simulink model "dual_arm_1"  (R2021b)
settings: Solver=FixedStepAuto  StartTime=0.0  StopTime=10  FixedStep=0.01  RelTol=1e-3
values from neighbouring files (symbols this model uses):
  a0 = 0.99    [load_main.m]
  b1 = base1.q    [load_main.m]
  b2 = base2.q    [load_main.m]
  berta = 0.98    [load_main.m]
  csi = 0.4    [load_main.m]
  dyr_in = [0 0 0 0 0 0]'    [load_main.m]
  F_int_max = [5;5]    [load_main.m]
  F_max = [1;1]    [load_main.m]
  franka_dh_matrix = [FEp_DH_theta;FEp_DH_d; FEp_DH_a;FEp_DH_alpha]    [load_main.m]
  inc = 1000    [load_main.m]
  mass = 1    [load_main.m]    (also in mod_k.m)
  q_in_1 = [0.4670   -0.1818    0.1521   -2.2022   -2.1767    2.4575    2.3293]    [load_main.m]
  q_in_2 = [-0.4654   -0.1791   -0.1528   -2.1994    2.1769    2.4577   -2.3291]    [load_main.m]
  Ts = 0.01    [load_main.m]
  yr_in = vec6(log(DQ(e_in)))    [load_main.m]
undefined symbols (not defined in the file or in its folder): k_default
settings Model: Creator=rachele  LastModifiedBy=geriatronics
settings SolverCC: AlgebraicLoopSolver=TrustRegion
settings DebuggingCC: SFMachineParentedDataDiag=warning

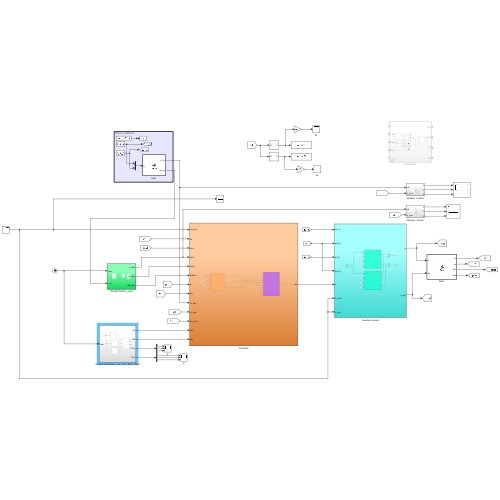
[thumbnail: Simulink's stored preview of the top-level diagram]
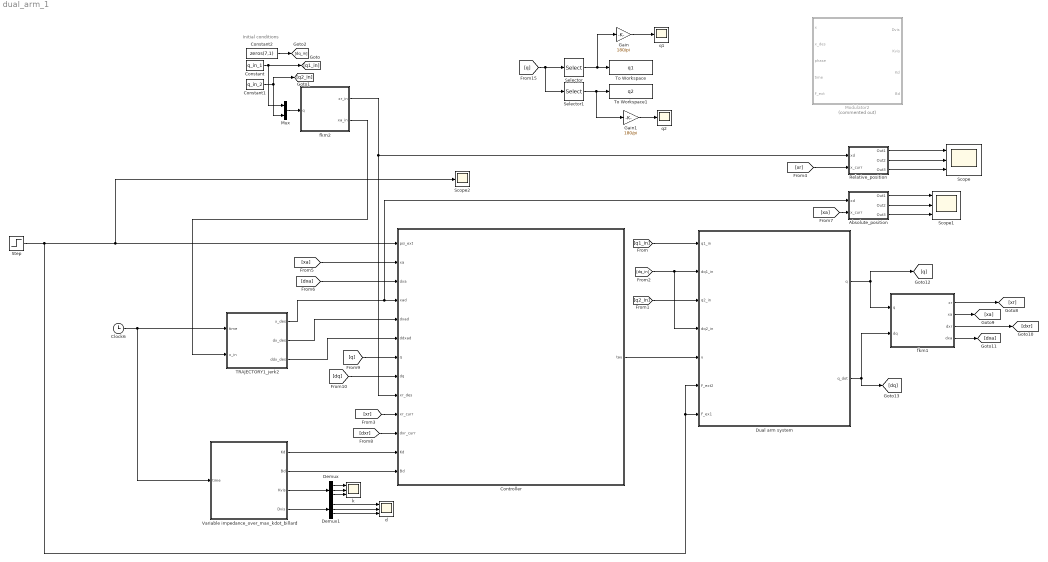
== system dual_arm_1 ==
  note: Initial conditions
  Absolute_position : Subsystem
  Clock6 : Clock
  Constant : Constant  Value=q_in_1
  Constant1 : Constant  Value=q_in_2
  Constant2 : Constant  Value=zeros(7,1)
  Controller : Subsystem
  Demux : Demux  Outputs=3
  Demux1 : Demux  Outputs=3
  Dual arm system : Subsystem
  Gain : Gain  Gain=180/pi
  Gain1 : Gain  Gain=180/pi
  Modulator2 : Subsystem  Commented=on
  Mux : Mux  Inputs=2
  Relative_position : Subsystem
  Scope : Scope  NumInputPorts=3
  Scope1 : Scope  NumInputPorts=3
  Scope2 : Scope
  Selector : Selector  InputPortWidth=14  IndexOptions=Index vector (dialog)  Indices=[1 2 3 4 5 6 7]  OutputSizes=1
  Selector1 : Selector  InputPortWidth=14  IndexOptions=Index vector (dialog)  Indices=[8 9 10 11 12 13 14]  OutputSizes=1
  Step : Step  After=[0;0;-1;0;0;0]*0  SampleTime=0
  TRAJECTORY1_jerk2 : Subsystem
  To Workspace : ToWorkspace  VariableName=q1  SaveFormat=Timeseries  SampleTime=-1
  To Workspace1 : ToWorkspace  VariableName=q2  SaveFormat=Timeseries  SampleTime=-1
  Variable impedance_over_max_kdot_billard : Subsystem
  d : Scope  NumInputPorts=3
  fkm1 : MATLAB Function  TreatAsAtomicUnit=on
  fkm2 : MATLAB Function  TreatAsAtomicUnit=on
  k : Scope  NumInputPorts=3
  q1 : Scope
  q2 : Scope
  wires:
  Constant/1 -> Mux/1, [q1_in]
  Constant1/1 -> Mux/2, [q2_in]
  Constant2/1 -> [dq_in]
  Clock6/1 -> Variable impedance_over_max_kdot_billard/1(time), TRAJECTORY1_jerk2/1(time)
  [q2_in] -> Dual arm system/3(q2_in)
  [q1_in] -> Dual arm system/1(q1_in)
  [dq_in] -> Dual arm system/4(dq2_in), Dual arm system/2(dq1_in)
  [q] -> Selector1/1, Selector/1
  Selector/1 -> Gain/1, To Workspace/1
  Selector1/1 -> Gain1/1, To Workspace1/1
  Gain/1 -> q1/1
  Gain1/1 -> q2/1
  Mux/1 -> fkm2/1(q)
  Dual arm system/2(q_dot) -> [dq], fkm1/2(dq)
  [q] -> Controller/7(q)
  [dq] -> Controller/8(dq)
  fkm1/4(dxa) -> [dxa]
  fkm1/3(dxr) -> [dxr]
  fkm1/2(xa) -> [xa]
  fkm1/1(xr) -> [xr]
  Controller/1(tau) -> Dual arm system/5(u)
  [xr] -> Relative_position/2(x_curr)
  Relative_position/1(Out1) -> Scope/1
  Relative_position/2(Out2) -> Scope/2
  Relative_position/3(Out3) -> Scope/3
  Absolute_position/1(Out1) -> Scope1/1
  Absolute_position/2(Out2) -> Scope1/2
  Absolute_position/3(Out3) -> Scope1/3
  TRAJECTORY1_jerk2/1(x_des) -> Absolute_position/1(xd), Controller/4(xad)
  TRAJECTORY1_jerk2/2(dx_des) -> Controller/5(dxad)
  TRAJECTORY1_jerk2/3(ddx_des) -> Controller/6(ddxad)
  [xa] -> Controller/2(xa)
  [dxa] -> Controller/3(dxa)
  fkm2/1(xr_in) -> Relative_position/1(xd), Controller/9(xr_des)
  [xa] -> Absolute_position/2(x_curr)
  fkm2/2(xa_in) -> TRAJECTORY1_jerk2/2(x_in)
  [xr] -> Controller/10(xr_curr)
  [dxr] -> Controller/11(dxr_curr)
  Dual arm system/1(q) -> fkm1/1(q), [q]
  Variable impedance_over_max_kdot_billard/1(Kd) -> Controller/12(Kd)
  Variable impedance_over_max_kdot_billard/2(Bd) -> Controller/13(Bd)
  Variable impedance_over_max_kdot_billard/3(Kvis) -> Demux/1
  Demux/1 -> k/1
  Demux/2 -> k/2
  Demux/3 -> k/3
  Variable impedance_over_max_kdot_billard/4(Dvis) -> Demux1/1
  Demux1/1 -> d/1
  Demux1/2 -> d/2
  Demux1/3 -> d/3
  Step/1 -> Dual arm system/6(F_ext2), Dual arm system/7(F_ex1), Controller/1(psi_ext), Scope2/1

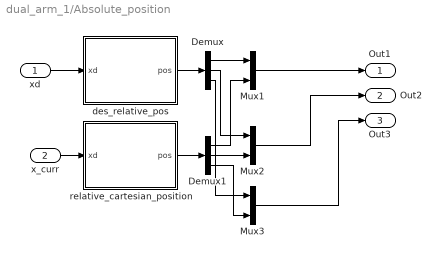
== system dual_arm_1/Absolute_position ==
  xd : Inport
  x_curr : Inport  Port=2
  Demux : Demux  Outputs=3
  Demux1 : Demux  Outputs=3
  Mux1 : Mux  Inputs=2
  Mux2 : Mux  Inputs=2
  Mux3 : Mux  Inputs=2
  des_relative_pos : MATLAB Function  TreatAsAtomicUnit=on
  relative_cartesian_position : MATLAB Function  TreatAsAtomicUnit=on
  Out1 : Outport
  Out2 : Outport  Port=2
  Out3 : Outport  Port=3
  wires:
  Demux/1 -> Mux1/1
  Demux1/1 -> Mux1/2
  Demux/3 -> Mux3/1
  des_relative_pos/1(pos) -> Demux/1
  Demux/2 -> Mux2/1
  xd/1 -> des_relative_pos/1(xd)
  Mux3/1 -> Out3/1
  Mux2/1 -> Out2/1
  Demux1/3 -> Mux3/2
  relative_cartesian_position/1(pos) -> Demux1/1
  x_curr/1 -> relative_cartesian_position/1(xd)
  Mux1/1 -> Out1/1
  Demux1/2 -> Mux2/2

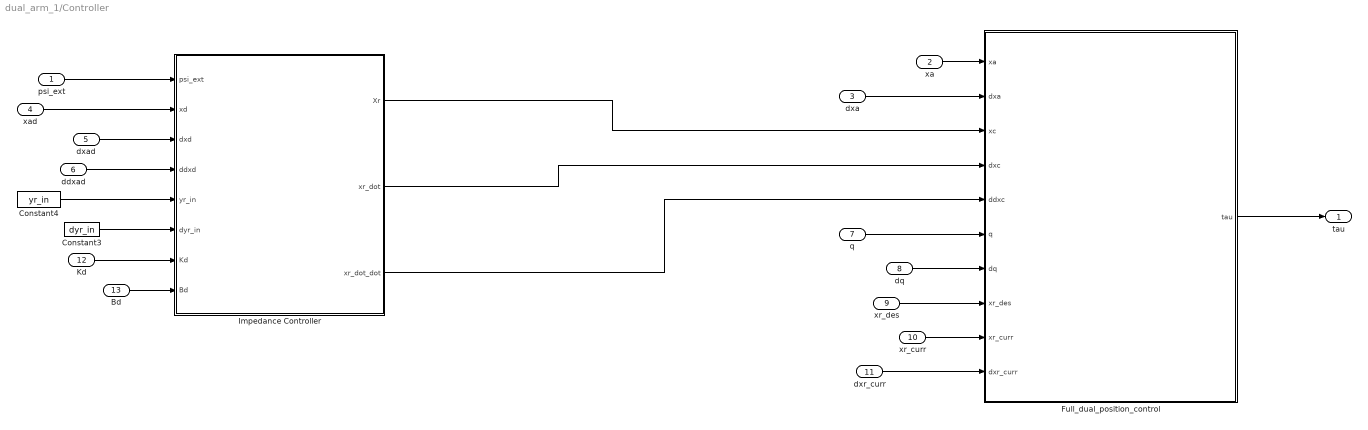
== system dual_arm_1/Controller ==
  psi_ext : Inport
  xa : Inport  Port=2
  dxa : Inport  Port=3
  xad : Inport  Port=4
  dxad : Inport  Port=5
  ddxad : Inport  Port=6
  q : Inport  Port=7
  dq : Inport  Port=8
  xr_des : Inport  Port=9
  xr_curr : Inport  Port=10
  dxr_curr : Inport  Port=11
  Kd : Inport  Port=12
  Bd : Inport  Port=13
  Constant3 : Constant  Value=dyr_in
  Constant4 : Constant  Value=yr_in
  Full_dual_position_control : Subsystem
  Impedance Controller : Subsystem
  tau : Outport
  wires:
  dxa/1 -> Full_dual_position_control/2(dxa)
  Constant3/1 -> Impedance Controller/6(dyr_in)
  Constant4/1 -> Impedance Controller/5(yr_in)
  Impedance Controller/2(xr_dot) -> Full_dual_position_control/4(dxc)
  xa/1 -> Full_dual_position_control/1(xa)
  Impedance Controller/3(xr_dot_dot) -> Full_dual_position_control/5(ddxc)
  Impedance Controller/1(Xr) -> Full_dual_position_control/3(xc)
  psi_ext/1 -> Impedance Controller/1(psi_ext)
  xad/1 -> Impedance Controller/2(xd)
  dxad/1 -> Impedance Controller/3(dxd)
  ddxad/1 -> Impedance Controller/4(ddxd)
  q/1 -> Full_dual_position_control/6(q)
  dq/1 -> Full_dual_position_control/7(dq)
  Kd/1 -> Impedance Controller/7(Kd)
  Bd/1 -> Impedance Controller/8(Bd)
  Full_dual_position_control/1(tau) -> tau/1
  xr_des/1 -> Full_dual_position_control/8(xr_des)
  xr_curr/1 -> Full_dual_position_control/9(xr_curr)
  dxr_curr/1 -> Full_dual_position_control/10(dxr_curr)

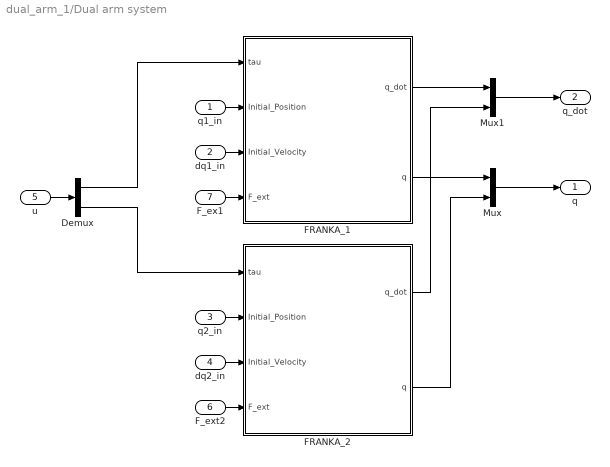
== system dual_arm_1/Dual arm system ==
  q1_in : Inport
  dq1_in : Inport  Port=2
  q2_in : Inport  Port=3
  dq2_in : Inport  Port=4
  u : Inport  Port=5
  F_ext2 : Inport  Port=6
  F_ex1 : Inport  Port=7
  Demux : Demux  Outputs=2
  FRANKA_1 : Subsystem
  FRANKA_2 : Subsystem
  Mux : Mux  Inputs=2
  Mux1 : Mux  Inputs=2
  q : Outport
  q_dot : Outport  Port=2
  wires:
  q2_in/1 -> FRANKA_2/2(Initial_Position)
  dq1_in/1 -> FRANKA_1/3(Initial_Velocity)
  q1_in/1 -> FRANKA_1/2(Initial_Position)
  F_ext2/1 -> FRANKA_2/4(F_ext)
  dq2_in/1 -> FRANKA_2/3(Initial_Velocity)
  F_ex1/1 -> FRANKA_1/4(F_ext)
  FRANKA_1/2(q) -> Mux/1
  FRANKA_2/2(q) -> Mux/2
  FRANKA_1/1(q_dot) -> Mux1/1
  FRANKA_2/1(q_dot) -> Mux1/2
  u/1 -> Demux/1
  Demux/1 -> FRANKA_1/1(tau)
  Demux/2 -> FRANKA_2/1(tau)
  Mux1/1 -> q_dot/1
  Mux/1 -> q/1

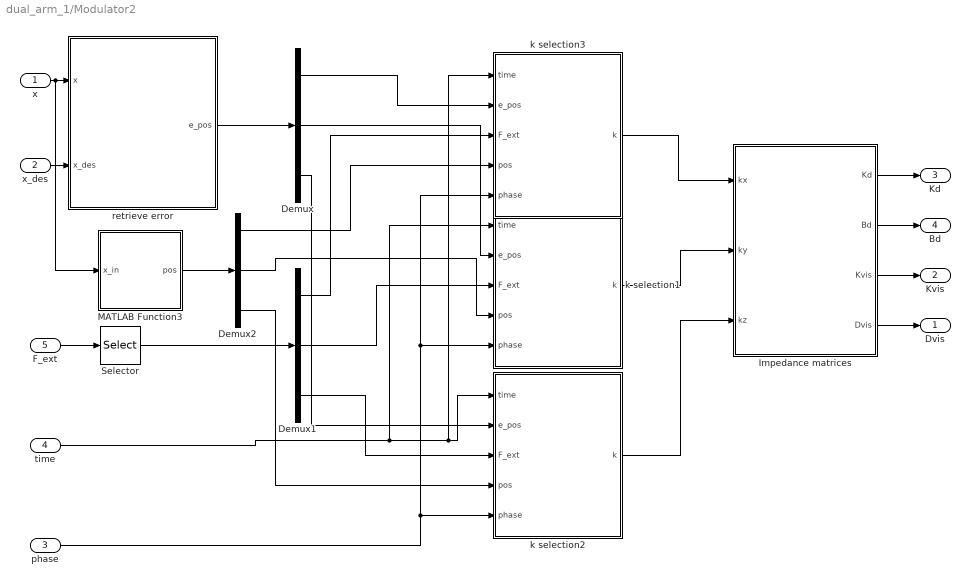
== system dual_arm_1/Modulator2 ==
  x : Inport
  x_des : Inport  Port=2
  phase : Inport  Port=3
  time : Inport  Port=4
  F_ext : Inport  Port=5
  Demux : Demux  Outputs=3
  Demux1 : Demux  Outputs=3
  Demux2 : Demux  Outputs=3
  Impedance matrices : MATLAB Function  TreatAsAtomicUnit=on
  MATLAB Function3 : MATLAB Function  TreatAsAtomicUnit=on
  Selector : Selector  InputPortWidth=6  IndexOptions=Index vector (dialog)  Indices=[1 2 3]  OutputSizes=1
  k selection1 : MATLAB Function  TreatAsAtomicUnit=on
  k selection2 : MATLAB Function  TreatAsAtomicUnit=on
  k selection3 : MATLAB Function  TreatAsAtomicUnit=on
  retrieve error : MATLAB Function  TreatAsAtomicUnit=on
  Dvis : Outport
  Kvis : Outport  Port=2
  Kd : Outport  Port=3
  Bd : Outport  Port=4
  wires:
  x_des/1 -> retrieve error/2(x_des)
  x/1 -> MATLAB Function3/1(x_in), retrieve error/1(x)
  F_ext/1 -> Selector/1
  retrieve error/1(e_pos) -> Demux/1
  k selection3/1(k) -> Impedance matrices/1(kx)
  Impedance matrices/1(Kd) -> Kd/1
  Impedance matrices/2(Bd) -> Bd/1
  Impedance matrices/3(Kvis) -> Kvis/1
  Impedance matrices/4(Dvis) -> Dvis/1
  Selector/1 -> Demux1/1
  MATLAB Function3/1(pos) -> Demux2/1
  phase/1 -> k selection2/5(phase), k selection1/5(phase), k selection3/5(phase)
  Demux1/2 -> k selection1/3(F_ext)
  Demux2/2 -> k selection1/4(pos)
  Demux/2 -> k selection1/2(e_pos)
  Demux2/1 -> k selection3/4(pos)
  Demux1/1 -> k selection3/3(F_ext)
  Demux/1 -> k selection3/2(e_pos)
  Demux/3 -> k selection2/2(e_pos)
  time/1 -> k selection1/1(time), k selection2/1(time), k selection3/1(time)
  k selection1/1(k) -> Impedance matrices/2(ky)
  Demux1/3 -> k selection2/3(F_ext)
  Demux2/3 -> k selection2/4(pos)
  k selection2/1(k) -> Impedance matrices/3(kz)

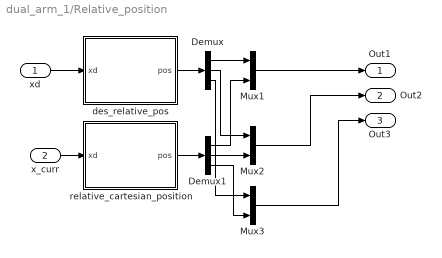
== system dual_arm_1/Relative_position ==
  xd : Inport
  x_curr : Inport  Port=2
  Demux : Demux  Outputs=3
  Demux1 : Demux  Outputs=3
  Mux1 : Mux  Inputs=2
  Mux2 : Mux  Inputs=2
  Mux3 : Mux  Inputs=2
  des_relative_pos : MATLAB Function  TreatAsAtomicUnit=on
  relative_cartesian_position : MATLAB Function  TreatAsAtomicUnit=on
  Out1 : Outport
  Out2 : Outport  Port=2
  Out3 : Outport  Port=3
  wires:
  Demux/1 -> Mux1/1
  Demux1/1 -> Mux1/2
  Demux/3 -> Mux3/1
  des_relative_pos/1(pos) -> Demux/1
  Demux/2 -> Mux2/1
  xd/1 -> des_relative_pos/1(xd)
  Mux3/1 -> Out3/1
  Mux2/1 -> Out2/1
  Demux1/3 -> Mux3/2
  relative_cartesian_position/1(pos) -> Demux1/1
  x_curr/1 -> relative_cartesian_position/1(xd)
  Mux1/1 -> Out1/1
  Demux1/2 -> Mux2/2

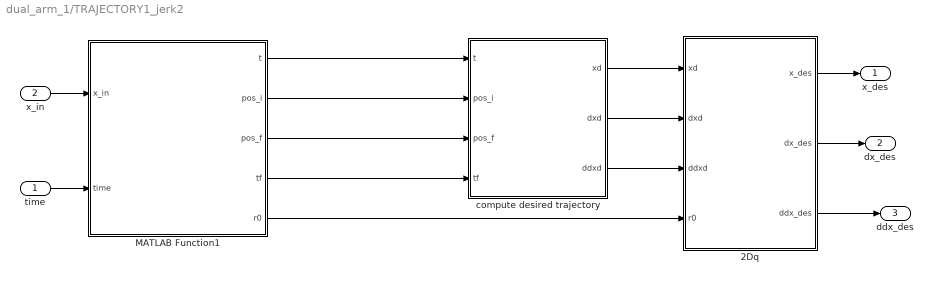
== system dual_arm_1/TRAJECTORY1_jerk2 ==
  time : Inport
  x_in : Inport  Port=2
  2Dq : MATLAB Function  TreatAsAtomicUnit=on
  MATLAB Function1 : MATLAB Function  TreatAsAtomicUnit=on
  compute desired trajectory : MATLAB Function  TreatAsAtomicUnit=on
  x_des : Outport
  dx_des : Outport  Port=2
  ddx_des : Outport  Port=3
  wires:
  compute desired trajectory/1(xd) -> 2Dq/1(xd)
  compute desired trajectory/2(dxd) -> 2Dq/2(dxd)
  compute desired trajectory/3(ddxd) -> 2Dq/3(ddxd)
  2Dq/1(x_des) -> x_des/1
  2Dq/2(dx_des) -> dx_des/1
  2Dq/3(ddx_des) -> ddx_des/1
  x_in/1 -> MATLAB Function1/1(x_in)
  time/1 -> MATLAB Function1/2(time)
  MATLAB Function1/1(t) -> compute desired trajectory/1(t)
  MATLAB Function1/2(pos_i) -> compute desired trajectory/2(pos_i)
  MATLAB Function1/3(pos_f) -> compute desired trajectory/3(pos_f)
  MATLAB Function1/4(tf) -> compute desired trajectory/4(tf)
  MATLAB Function1/5(r0) -> 2Dq/4(r0)

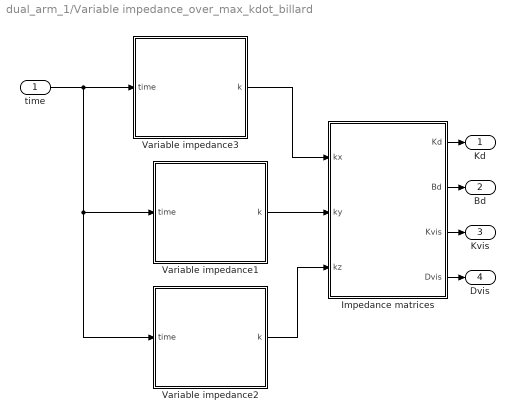
== system dual_arm_1/Variable impedance_over_max_kdot_billard ==
  time : Inport
  Impedance matrices : MATLAB Function  TreatAsAtomicUnit=on
  Variable impedance1 : MATLAB Function  TreatAsAtomicUnit=on
  Variable impedance2 : MATLAB Function  TreatAsAtomicUnit=on
  Variable impedance3 : MATLAB Function  TreatAsAtomicUnit=on
  Kd : Outport
  Bd : Outport  Port=2
  Kvis : Outport  Port=3
  Dvis : Outport  Port=4
  wires:
  Impedance matrices/4(Dvis) -> Dvis/1
  Variable impedance1/1(k) -> Impedance matrices/2(ky)
  Impedance matrices/1(Kd) -> Kd/1
  time/1 -> Variable impedance3/1(time), Variable impedance2/1(time), Variable impedance1/1(time)
  Variable impedance2/1(k) -> Impedance matrices/3(kz)
  Variable impedance3/1(k) -> Impedance matrices/1(kx)
  Impedance matrices/2(Bd) -> Bd/1
  Impedance matrices/3(Kvis) -> Kvis/1

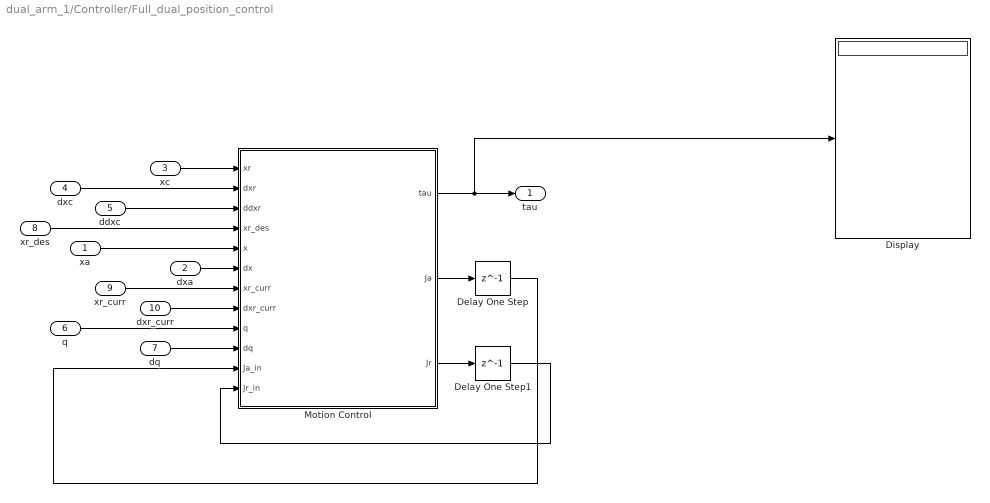
== system dual_arm_1/Controller/Full_dual_position_control ==
  xa : Inport
  dxa : Inport  Port=2
  xc : Inport  Port=3
  dxc : Inport  Port=4
  ddxc : Inport  Port=5
  q : Inport  Port=6
  dq : Inport  Port=7
  xr_des : Inport  Port=8
  xr_curr : Inport  Port=9
  dxr_curr : Inport  Port=10
  Delay One Step : Delay  DelayLength=1
  Delay One Step1 : Delay  DelayLength=1
  Display : Display
  Motion Control : MATLAB Function  TreatAsAtomicUnit=on
  tau : Outport
  wires:
  Motion Control/1(tau) -> Display/1, tau/1
  dxa/1 -> Motion Control/6(dx)
  ddxc/1 -> Motion Control/3(ddxr)
  q/1 -> Motion Control/9(q)
  dxc/1 -> Motion Control/2(dxr)
  xa/1 -> Motion Control/5(x)
  dq/1 -> Motion Control/10(dq)
  xc/1 -> Motion Control/1(xr)
  xr_des/1 -> Motion Control/4(xr_des)
  xr_curr/1 -> Motion Control/7(xr_curr)
  dxr_curr/1 -> Motion Control/8(dxr_curr)
  Motion Control/2(Ja) -> Delay One Step/1
  Motion Control/3(Jr) -> Delay One Step1/1
  Delay One Step1/1 -> Motion Control/12(Jr_in)
  Delay One Step/1 -> Motion Control/11(Ja_in)

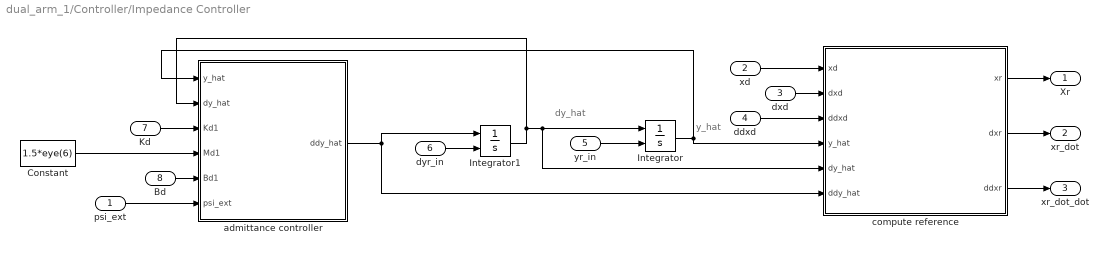
== system dual_arm_1/Controller/Impedance Controller ==
  note: y_hat
  note: dy_hat
  psi_ext : Inport
  xd : Inport  Port=2
  dxd : Inport  Port=3
  ddxd : Inport  Port=4
  yr_in : Inport  Port=5
  dyr_in : Inport  Port=6
  Kd : Inport  Port=7
  Bd : Inport  Port=8
  Constant : Constant  Value=1.5*eye(6)
  Integrator : Integrator  InitialConditionSource=external
  Integrator1 : Integrator  InitialConditionSource=external
  admittance controller : MATLAB Function  TreatAsAtomicUnit=on
  compute reference : MATLAB Function  TreatAsAtomicUnit=on
  Xr : Outport
  xr_dot : Outport  Port=2
  xr_dot_dot : Outport  Port=3
  wires:
  admittance controller/1(ddy_hat) -> Integrator1/1, compute reference/6(ddy_hat)
  Integrator1/1 -> admittance controller/2(dy_hat), compute reference/5(dy_hat), Integrator/1
  dxd/1 -> compute reference/2(dxd)
  xd/1 -> compute reference/1(xd)
  psi_ext/1 -> admittance controller/6(psi_ext)
  ddxd/1 -> compute reference/3(ddxd)
  compute reference/1(xr) -> Xr/1
  compute reference/2(dxr) -> xr_dot/1
  compute reference/3(ddxr) -> xr_dot_dot/1
  Integrator/1 -> admittance controller/1(y_hat), compute reference/4(y_hat)
  yr_in/1 -> Integrator/2
  dyr_in/1 -> Integrator1/2
  Kd/1 -> admittance controller/3(Kd1)
  Constant/1 -> admittance controller/4(Md1)
  Bd/1 -> admittance controller/5(Bd1)

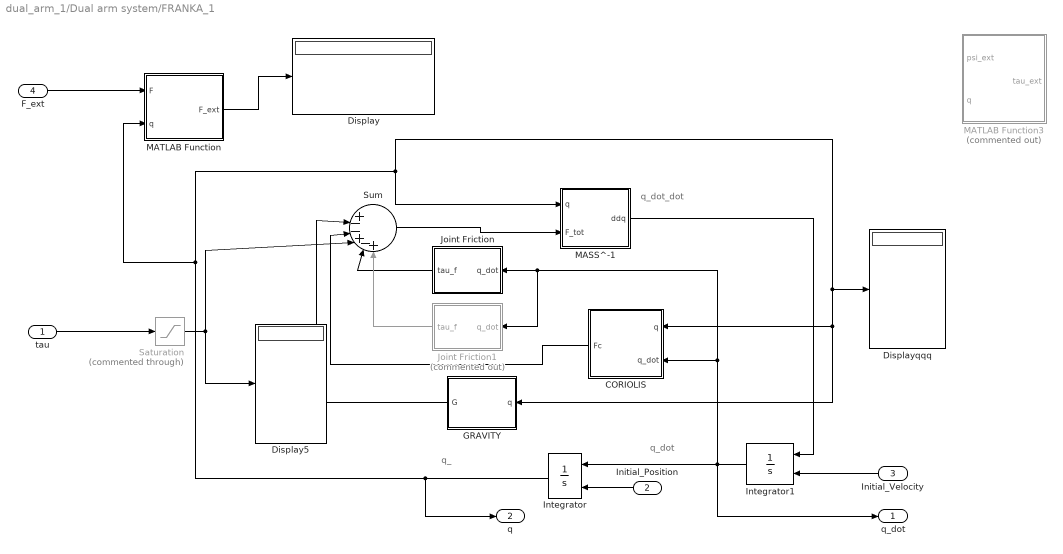
== system dual_arm_1/Dual arm system/FRANKA_1 ==
  note: q_dot
  note: q_dot_dot
  note: q_
  tau : Inport
  Initial_Position : Inport  Port=2
  Initial_Velocity : Inport  Port=3
  F_ext : Inport  Port=4
  CORIOLIS : MATLAB Function  TreatAsAtomicUnit=on
  Display : Display
  Display5 : Display
  Displayqqq : Display
  GRAVITY : MATLAB Function  TreatAsAtomicUnit=on
  Integrator : Integrator  InitialConditionSource=external
  Integrator1 : Integrator  InitialConditionSource=external  InitialCondition=[0;0]
  Joint Friction : MATLAB Function  TreatAsAtomicUnit=on
  Joint Friction1 : MATLAB Function  Commented=on  TreatAsAtomicUnit=on
  MASS^-1 : MATLAB Function  TreatAsAtomicUnit=on
  MATLAB Function : MATLAB Function  TreatAsAtomicUnit=on
  MATLAB Function3 : MATLAB Function  Commented=on  TreatAsAtomicUnit=on
  Saturation : Saturate  Commented=through  UpperLimit=100  LowerLimit=-100
  Sum : Sum  Inputs=||+--+-+
  q_dot : Outport
  q : Outport  Port=2
  wires:
  GRAVITY/1(G) -> Sum/2
  Initial_Position/1 -> Integrator/2
  Integrator/1 -> MATLAB Function/2(q), MASS^-1/1(q), GRAVITY/1(q), CORIOLIS/1(q), Displayqqq/1, q/1
  Integrator1/1 -> q_dot/1, CORIOLIS/2(q_dot), Joint Friction1/1(q_dot), Joint Friction/1(q_dot), Integrator/1
  Initial_Velocity/1 -> Integrator1/2
  MASS^-1/1(ddq) -> Integrator1/1
  Sum/1 -> MASS^-1/2(F_tot)
  CORIOLIS/1(Fc) -> Sum/3
  tau/1 -> Saturation/1
  Joint Friction/1(tau_f) -> Sum/5
  Joint Friction1/1(tau_f) -> Sum/6
  Saturation/1 -> Display5/1, Sum/4
  F_ext/1 -> MATLAB Function/1(F)
  MATLAB Function/1(F_ext) -> Display/1

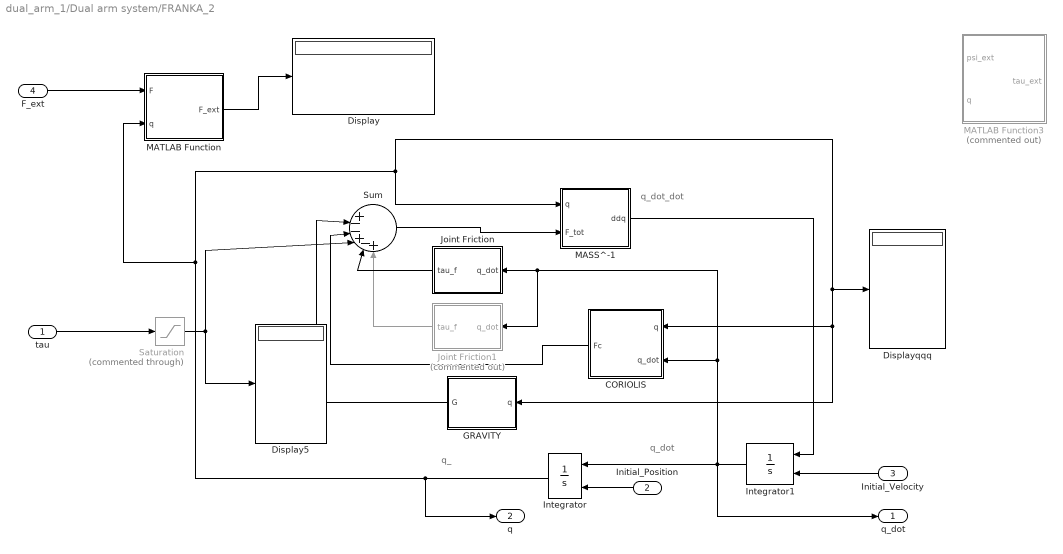
== system dual_arm_1/Dual arm system/FRANKA_2 ==
  note: q_
  note: q_dot_dot
  note: q_dot
  tau : Inport
  Initial_Position : Inport  Port=2
  Initial_Velocity : Inport  Port=3
  F_ext : Inport  Port=4
  CORIOLIS : MATLAB Function  TreatAsAtomicUnit=on
  Display : Display
  Display5 : Display
  Displayqqq : Display
  GRAVITY : MATLAB Function  TreatAsAtomicUnit=on
  Integrator : Integrator  InitialConditionSource=external
  Integrator1 : Integrator  InitialConditionSource=external  InitialCondition=[0;0]
  Joint Friction : MATLAB Function  TreatAsAtomicUnit=on
  Joint Friction1 : MATLAB Function  Commented=on  TreatAsAtomicUnit=on
  MASS^-1 : MATLAB Function  TreatAsAtomicUnit=on
  MATLAB Function : MATLAB Function  TreatAsAtomicUnit=on
  MATLAB Function3 : MATLAB Function  Commented=on  TreatAsAtomicUnit=on
  Saturation : Saturate  Commented=through  UpperLimit=100  LowerLimit=-100
  Sum : Sum  Inputs=||+--+-+
  q_dot : Outport
  q : Outport  Port=2
  wires:
  MATLAB Function/1(F_ext) -> Display/1
  F_ext/1 -> MATLAB Function/1(F)
  Saturation/1 -> Sum/4, Display5/1
  Joint Friction1/1(tau_f) -> Sum/6
  Joint Friction/1(tau_f) -> Sum/5
  tau/1 -> Saturation/1
  CORIOLIS/1(Fc) -> Sum/3
  Sum/1 -> MASS^-1/2(F_tot)
  MASS^-1/1(ddq) -> Integrator1/1
  Initial_Velocity/1 -> Integrator1/2
  Integrator1/1 -> Integrator/1, Joint Friction/1(q_dot), Joint Friction1/1(q_dot), CORIOLIS/2(q_dot), q_dot/1
  Integrator/1 -> q/1, Displayqqq/1, CORIOLIS/1(q), GRAVITY/1(q), MASS^-1/1(q), MATLAB Function/2(q)
  Initial_Position/1 -> Integrator/2
  GRAVITY/1(G) -> Sum/2

== matlab function dual_arm_1/Relative_position/des_relative_pos ==
  data: xd input; pos output
function pos  = fcn(xd)
coder.extrinsic('DQ','vec4','translation');
%retrieve position, rotation axis and angle
y = zeros(4,1);
pos = zeros(3,1);
y = vec4(translation(DQ(xd)));
pos = [y(2);y(3);y(4)];
end

== matlab function dual_arm_1/Absolute_position/des_relative_pos ==
  data: xd input; pos output
function pos  = fcn(xd)
coder.extrinsic('DQ','vec4','translation');
%retrieve position, rotation axis and angle
y = zeros(4,1);
pos = zeros(3,1);
y = vec4(translation(DQ(xd)));
pos = [y(2);y(3);y(4)];
end

== matlab function dual_arm_1/Relative_position/relative_cartesian_position ==
  data: xd input; pos output
function pos  = fcn(xd)
coder.extrinsic('DQ','vec4','translation');
%retrieve position, rotation axis and angle
y = zeros(4,1);
pos = zeros(3,1);
y = vec4(translation(DQ(xd)));
pos = [y(2);y(3);y(4)];
end

== matlab function dual_arm_1/Absolute_position/relative_cartesian_position ==
  data: xd input; pos output
function pos  = fcn(xd)
coder.extrinsic('DQ','vec4','translation');
%retrieve position, rotation axis and angle
y = zeros(4,1);
pos = zeros(3,1);
y = vec4(translation(DQ(xd)));
pos = [y(2);y(3);y(4)];
end

== matlab function dual_arm_1/Modulator2/Impedance matrices ==
  data: kx input; Kd output; ky input; kz input; Bd output; Kvis output; Dvis output; mass parameter
function [Kd,Bd,Kvis,Dvis] = fcn(kx,ky,kz,mass)
%% Final impedance matrices

% damping computation, (critically damped condition)
dx = sqrt(4*kx*mass)*4;
dy = sqrt(4*ky*mass)*4;
dz = sqrt(4*kz*mass)*4;

%% Final impedance matrices
Bd = zeros(6,6);
Kd = zeros(6,6);
Bd(4:6,4:6) = diag([dx, dy, dz]);
Bd(1:3,1:3) = diag([2*sqrt(300) 2*sqrt(300) 2*sqrt(300)]); %rot damping
Kd(4:6,4:6) = diag([kx, ky, kz]);
Kd(1:3,1:3) = diag ([300 300 300]); %rot stiffness
% Kd = 300*eye(6);
% Bd = 50*eye(6); 
Kvis = [kx; ky; kz];
Dvis = [dx; dy; dz];
end

== matlab function dual_arm_1/Variable impedance_over_max_kdot_billard/Impedance matrices ==
  data: kx input; Kd output; ky input; kz input; Bd output; Kvis output; Dvis output
function [Kd,Bd,Kvis,Dvis] = fcn(kx,ky,kz)
%% Final impedance matrices
mass = 1; 

% damping computation, (critically damped condition)
dx = sqrt(4*kx*mass);
dy = sqrt(4*ky*mass);
dz = sqrt(4*kz*mass);

%% Final impedance matrices
Bd = zeros(6,6);
Kd = zeros(6,6);

Kd = diag([kx;ky;kz;kx;ky;kz]);
Bd = diag([dx;dy;dz;dx;dy;dz]); 


Kvis = [kx; ky; kz];
Dvis = [dx; dy; dz];
end

== matlab function dual_arm_1/Variable impedance_over_max_kdot_billard/Variable impedance3 ==
  settings: updateMethod=DISCRETE  sampleTime=0.01
  data: time input; k output; berta parameter; csi parameter; a0 parameter; inc parameter
function k = fcn(time, berta, csi, a0, inc)

%% change gains on each dof separately

%%Paramters
k_max = 10000; %N/m
mass = 1; %kg

%% Initialization
persistent ki  time_prec

% persistent initialization
if isempty(ki)
    ki = 100;
end

if isempty(time_prec)
    time_prec = 0;
end

k_dot = 10*berta*(4*a0*sqrt(ki/mass)*(ki)^(3/2))/(sqrt(ki) + 2*a0*csi*sqrt(ki)); %maximum variation within stability conditions 
k_temp = ki + inc*k_dot*(time -time_prec);

if k_temp >= k_max
    ki = k_max;
else
    ki = k_temp;
end

k = ki;


time_prec = time; 

end

== matlab function dual_arm_1/Variable impedance_over_max_kdot_billard/Variable impedance1 ==
  settings: updateMethod=DISCRETE  sampleTime=0.01
  data: time input; k output; berta parameter; csi parameter; a0 parameter; inc parameter
function k = fcn(time, berta, csi, a0, inc)

%% change gains on each dof separately

%%Paramters
k_max = 10000; %N/m
mass = 1; %kg

%% Initialization
persistent ki  time_prec

% persistent initialization
if isempty(ki)
    ki = 100;
end

if isempty(time_prec)
    time_prec = 0;
end

k_dot = 10*berta*(4*a0*sqrt(ki/mass)*(ki)^(3/2))/(sqrt(ki) + 2*a0*csi*sqrt(ki)); %maximum variation within stability conditions 
k_temp = ki + inc*k_dot*(time -time_prec);

if k_temp >= k_max
    ki = k_max;
else
    ki = k_temp;
end

k = ki;


time_prec = time; 

end

== matlab function dual_arm_1/Variable impedance_over_max_kdot_billard/Variable impedance2 ==
  settings: updateMethod=DISCRETE  sampleTime=0.01
  data: time input; k output; berta parameter; csi parameter; a0 parameter; inc parameter
function k = fcn(time, berta, csi, a0, inc)

%% change gains on each dof separately

%%Paramters
k_max = 10000; %N/m
mass = 1; %kg

%% Initialization
persistent ki  time_prec

% persistent initialization
if isempty(ki)
    ki = 100;
end

if isempty(time_prec)
    time_prec = 0;
end

k_dot = 10*berta*(4*a0*sqrt(ki/mass)*(ki)^(3/2))/(sqrt(ki) + 2*a0*csi*sqrt(ki)); %maximum variation within stability conditions 
k_temp = ki + inc*k_dot*(time -time_prec);

if k_temp >= k_max
    ki = k_max;
else
    ki = k_temp;
end

k = ki;


time_prec = time; 

end

== matlab function dual_arm_1/Dual arm system/FRANKA_1/GRAVITY ==
  data: q input; G output double
function G = fcn(q)
coder.extrinsic('get_GravityVector');
G = zeros(7,1);
G = get_GravityVector(q);

end

== matlab function dual_arm_1/Dual arm system/FRANKA_1/MASS^-1 ==
  data: q input; ddq output; F_tot input double
function ddq = fcn(q,F_tot)
coder.extrinsic('get_MassMatrix');
B = zeros(7,7);
B = get_MassMatrix(q);
B(isnan(B)) = 0;

ddq = B\F_tot;                      % Ftot*M^-1

end

== matlab function dual_arm_1/Dual arm system/FRANKA_1/MATLAB Function3 ==
  data: psi_ext input; tau_ext output double; q input; franka_dh_matrix parameter
function tau_ext = fcn(psi_ext,q,franka_dh_matrix)
%% Description: maps external wrench into joint-space
coder.extrinsic('DQ','vec8'); 
coder.extrinsic('pose_jacobian','fkm','DQ_SerialManipulator');             
franka = DQ_SerialManipulator(franka_dh_matrix,'modified'); 
%% initialization
G = zeros(8,8);
J = zeros(8,8);
Jg = zeros(6,7); %geometric jacobian
x_pose = zeros(8,1);
tau_ext = zeros(7,1); 
%% fkm
x_pose = vec8(fkm(franka,[q;0]));
J = pose_jacobian(franka,[q;0]);
J1 = J(:,1:7); 
G = getG(x_pose); %generalized dual jacobian
Ibar = [zeros(3,1), eye(3), zeros(3,1), zeros(3,3);...
        zeros(3,1), zeros(3,3), zeros(3,1), eye(3)]; 
Jg = Ibar*G*J1;
tau_ext = (Jg)'* psi_ext;
end

== matlab function dual_arm_1/Dual arm system/FRANKA_1/MATLAB Function ==
  data: F input; F_ext output double; q input
function F_ext  = fcn(F,q)
coder.extrinsic('loadrobot','geometricJacobian');
franka_cfr = loadrobot("frankaEmikaPanda", "DataFormat","row");
%init
F_ext = zeros(7,1);
Jg1 = zeros(6,9);
%get numeric geometric jacobian
Jg1 = geometricJacobian(franka_cfr,[q',0,0],'panda_link8');
Jg = Jg1(:,1:7);
Jg = [Jg(4:6,:);Jg(1:3,:)]; 
F_ext = (Jg')*F;

end

== matlab function dual_arm_1/Controller/Impedance Controller/admittance controller ==
  settings: sampleTime=Ts
  data: y_hat input; ddy_hat output; dy_hat input; Kd1 input; Md1 input; Bd1 input; psi_ext input

function ddy_hat = adm_contr(y_hat,dy_hat,Kd1,Md1,Bd1,psi_ext)
%% Description: admittance controller to enforce an apparent impedance behaviour at task-space
coder.extrinsic('get_Glog','getG','getQ8');
coder.extrinsic('DQ','vec8','vec6','vec4','P','D','hamiplus8','plus','minus','mtimes','log','exp');
%initialization
Glog = zeros(6,6);
ddy_hat = zeros(6,1); 
x_hat = zeros(8,1); 
Q8 = zeros(8,6);
G = zeros(8,8); 
%retrieve utils
Ibar = [zeros(3,1), eye(3), zeros(3,1), zeros(3,3);...
        zeros(3,1), zeros(3,3), zeros(3,1), eye(3)];
x_hat = vec8(exp(DQ(y_hat))); %pose displacement 
% Glog = get_Glog(x_hat);
G = getG(DQ(x_hat));
Q8 = getQ8(DQ(x_hat));
Glog = Ibar*G*Q8;
flog = (Glog)'*(psi_ext); %external wrench consistent with log mapping

%% admittance equation
% ddy_hat = inv(Md1)*(-Bd1*dy_hat-Kd1*y_hat-flog); 

ddy_hat = inv(Md1)*(-Bd1*dy_hat-Kd1*y_hat-flog); 
end

== matlab function dual_arm_1/Controller/Impedance Controller/compute reference ==
  settings: sampleTime=Ts
  data: xr output; dxr output; xd input; dxd input; ddxd input; ddxr output; y_hat input; dy_hat input; ddy_hat input; C8 parameter
function [xr,dxr,ddxr] = cp_ref(xd,dxd,ddxd,y_hat,dy_hat,ddy_hat,C8)
%% description: impedance control law to enforce virtual desired impedance
%compute references xr,dxr,ddxr to guarantee compliant behaviour to be given to
%to the inner motion loop.

%inputs:  xd,dxd,ddxd = desired pose variable;
%         y_hat,dy_hat,ddy_hat = logarithm mapping of displacement error
%         between xd and xr
%       
%outputs: xr,dxr,ddxr = reference for inner motion loop 

coder.extrinsic('getQ8','getQ8_dot');
coder.extrinsic('DQ','vec8','vec6','vec4','P','D','hamiplus4','haminus4','haminus8','norm','hamiplus8','translation','rotation_angle','rotation_axis','plus','minus','mtimes','log','exp');

%% initialization
Q8 = zeros(8,6);
Q8_dot = zeros(8,6);
xr = zeros(8,1);
dxr = zeros(8,1);
ddxr = zeros(8,1); 

%compute displacement between desired and reference pose  
x_hat = vec8(exp(DQ(y_hat)));
Q8 = getQ8(DQ(x_hat)); 
dx_hat = Q8*dy_hat;
Q8_dot = getQ8_dot(DQ(x_hat),DQ(dx_hat)); 
ddx_hat = Q8*ddy_hat + Q8_dot*dy_hat; 
%retrieve reference
xr = hamiplus8(DQ(xd))*C8*x_hat;
dxr = hamiplus8(DQ(dxd))*C8*x_hat + hamiplus8(DQ(xd))*C8*dx_hat;
ddxr = hamiplus8(DQ(ddxd))*C8*x_hat + 2*hamiplus8(DQ(dxd))*C8*dx_hat + hamiplus8(DQ(xd))*C8*ddx_hat;

end

== matlab function dual_arm_1/Controller/Full_dual_position_control/Motion Control ==
  settings: sampleTime=Ts
  data: xr input; tau output; dxr input; ddxr input; xr_des input; x input; dx input; xr_curr input; dxr_curr input; q input; dq input; Ja_in input; Jr_in input; franka_dh_matrix parameter; b1 parameter; b2 parameter; Ja output; Jr output; Ts parameter
function [tau, Ja, Jr] = fcn(xr, dxr, ddxr, xr_des, x, dx, xr_curr, dxr_curr, q, dq, Ja_in, Jr_in, franka_dh_matrix, b1, b2, Ts)
%% Motion control: computes torque to track reference from admittance law.
%% FULL DUAL POSITION CONTROL
%% Task-space inverse dynamics with fb linearization: tau = M*y + C*dq * g * fric; 
%Inputs : xr,dxr,ddxr = dual reference position for absolute pose and its derivatives
%         xr_des = desired relative pose          
%         q,dq = joint angles and velocities
%         x,dx = current absolute pose
%         xr_curr,dx_curr = current relative pose
%Outpuy : tau = torque vector (7x1) joint-space

coder.extrinsic('DQ_SerialManipulator','DQ_CooperativeDualTaskSpace','relative_pose_jacobian','absolute_pose_jacobian','fkm','set_reference_frame');
coder.extrinsic('DQ','haminus8','plus','minus','mtimes','ctranspose');
coder.extrinsic('get_MassMatrix','get_GravityVector','get_CoriolisMatrix','get_FrictionTorque');

%% Initialization
M1 = zeros(7,7);
M2 = M1;
C1 = zeros(7,7);
C2 = C1; 
g1 = zeros(7,1);
g2 = g1; 
Jr = zeros(8,14);
Ja = zeros(8,14); 
fric1 = zeros(7,1);
fric2 = fric1; 
tau = zeros(14,1); 

%% Load robot
franka1 = DQ_SerialManipulator(franka_dh_matrix,'standard'); 
franka2 = DQ_SerialManipulator(franka_dh_matrix,'standard');
% set base reference
set_reference_frame(franka1,DQ(b1));
set_reference_frame(franka2,DQ(b2));
%dual-arm
two_arms =  DQ_CooperativeDualTaskSpace(franka1, franka2);

%get joint angles
q1 = q(1:7);
q2 = q(8:14);
dq1 = dq(1:7);
dq2 = dq(8:14); 

%% define augmented error (16x1)
er = xr_des - xr_curr; %relative pose error
ea = xr - x; %absolute pose error
e_tot = [er;ea];
der = -dxr_curr; 
dea = dxr - dx; 
de_tot = [der;dea]; 

%% Task-space inverse dynamics with feedback linearization
Kd = 5;
Kp = 20;

%get model matrices
M1 = get_MassMatrix(q1);
C1 = get_CoriolisMatrix(q1,dq1);
g1 = get_GravityVector(q1);
fric1 = get_FrictionTorque(dq1);
M2 = get_MassMatrix(q2);
C2 = get_CoriolisMatrix(q2,dq2);
g2 = get_GravityVector(q2);
fric2 = get_FrictionTorque(dq2);

M = blkdiag(M1,M2);
C = blkdiag(C1,C2);
g = [g1;g2];
fric = [fric1;fric2]; 

%get Jacobians
Jr = relative_pose_jacobian(two_arms,q);
Ja = absolute_pose_jacobian(two_arms,q); 
J_aug = [Jr;Ja];

%get Jacobian derivatives
Jr_dot = (Jr-Jr_in)/Ts; 
Ja_dot = (Ja-Ja_in)/Ts; 
J_dot = [Jr_dot;Ja_dot]; 

%% Control law (1.Task-space inverse dynamics with fb lin)

ddxd_aug = [zeros(8,1); ddxr]; 
ax = ddxd_aug - J_dot*dq + Kp*e_tot + Kd*de_tot; 
J_inv = pinv(J_aug); 
aq = J_inv*ax; 
tau = M*aq + C*dq + g + fric;

== matlab function dual_arm_1/Dual arm system/FRANKA_1/CORIOLIS ==
  data: q input; Fc output double; q_dot input
function Fc = fcn(q,q_dot)
coder.extrinsic('get_CoriolisMatrix');
C = zeros(7,7);
C = get_CoriolisMatrix(q,q_dot);

Fc = C*q_dot;

end

== matlab function dual_arm_1/Dual arm system/FRANKA_1/Joint Friction ==
  data: q_dot input; tau_f output
function tau_f = fcn(q_dot)
coder.extrinsic('get_FrictionTorque');
tau_f = zeros(7,1);
tau_f = get_FrictionTorque(q_dot);

end

== matlab function dual_arm_1/Dual arm system/FRANKA_1/Joint Friction1 ==
  data: q_dot input; tau_f output
function tau_f = fcn(q_dot)
D=eye(7)*1;
tau_f = -D*q_dot;

end

== matlab function dual_arm_1/Modulator2/MATLAB Function3 ==
  data: x_in input; pos output
function pos  = fcn(x_in)
coder.extrinsic('DQ','vec4','translation');
%% retrieve positio
y = zeros(4,1);
pos = zeros(3,1);
%pos 
y = vec4(translation(DQ(x_in)));
pos = [y(2);y(3);y(4)];
end

== matlab function dual_arm_1/Modulator2/k selection1 ==
  settings: updateMethod=DISCRETE
  data: time input; e_pos input; k output; F_ext input; F_max parameter; F_int_max parameter; k_default parameter; pos input; phase input; inc parameter; a0 parameter; berta parameter; csi parameter; mass parameter
function k = fcn(time,e_pos,F_ext,F_max, F_int_max,k_default,pos,phase,inc,a0, berta, csi,mass)

%% Description: Modulate stiffness and damping consequently of the admittance controller.
%%Inputs:     e_pos = position error 
%             F_ext = external force on EE
%             phase = flag acknowledging the current desired trajectory phase
%%Outputs:    k = value of stiffnes on single d.o.f
%%Parameters: F_max = treshold of disturbance
%             F_int_max = maximum interaction force
%             k_default = default value of stiffness
%             a0,berta,csi = parameters from stability conditions
%             mass = apparent mass

%% Initialization
persistent ki int time_prec

% persistent initialization
if isempty(ki)
    ki = k_default;
end

if isempty(int)
    int = 1000;
end

if isempty(time_prec)
    time_prec = 0;
end


%% Compute k
if phase == 0
    if abs(F_ext) > F_max %contact is detected
        ki = 0.995*ki;
        if int == 1000 %contact position not set yet
            int = pos;
        end
        % if interaction force is higher than threshold
        if ki*abs(e_pos) > F_int_max
            % set k
            ktemp_x = F_int_max/abs(e_pos);
            if ktemp_x < ki
                ki = ktemp_x;
            end
        end
    end
else
    if pos > int + 0.005 %safe to increase k
        k_dot = berta*(4*a0*sqrt(ki/mass)*(ki)^(3/2))/(sqrt(ki) + 2*a0*csi*sqrt(ki)); %maximum variation within stability conditions 
        k_tempx = ki + k_dot*(time -time_prec);
        %ki = inc*ki;
        ki = k_tempx;
        %if ki > k_default
        if k_tempx > k_default
            ki = k_default;
        end
    end
end

k = ki;
time_prec = time;
end

== matlab function dual_arm_1/Modulator2/k selection2 ==
  settings: updateMethod=DISCRETE
  data: time input; e_pos input; k output; F_ext input; F_max parameter; F_int_max parameter; k_default parameter; pos input; phase input; inc parameter; a0 parameter; berta parameter; csi parameter; mass parameter
function k = fcn(time,e_pos,F_ext,F_max, F_int_max,k_default,pos,phase,inc,a0, berta, csi,mass)

%% Description: Modulate stiffness and damping consequently of the admittance controller.
%%Inputs:     e_pos = position error 
%             F_ext = external force on EE
%             phase = flag acknowledging the current desired trajectory phase
%%Outputs:    k = value of stiffnes on single d.o.f
%%Parameters: F_max = treshold of disturbance
%             F_int_max = maximum interaction force
%             k_default = default value of stiffness
%             a0,berta,csi = parameters from stability conditions
%             mass = apparent mass

%% Initialization
persistent ki int time_prec

% persistent initialization
if isempty(ki)
    ki = k_default;
end

if isempty(int)
    int = 1000;
end

if isempty(time_prec)
    time_prec = 0;
end


%% Compute k
if phase == 0
    if abs(F_ext) > F_max %contact is detected
        ki = 0.995*ki;
        if int == 1000 %contact position not set yet
            int = pos;
        end
        % if interaction force is higher than threshold
        if ki*abs(e_pos) > F_int_max
            % set k
            ktemp_x = F_int_max/abs(e_pos);
            if ktemp_x < ki
                ki = ktemp_x;
            end
        end
    end
else
    if pos > int + 0.005 %safe to increase k
        k_dot = berta*(4*a0*sqrt(ki/mass)*(ki)^(3/2))/(sqrt(ki) + 2*a0*csi*sqrt(ki)); %maximum variation within stability conditions 
        k_tempx = ki + k_dot*(time -time_prec);
        %ki = inc*ki;
        ki = k_tempx;
        %if ki > k_default
        if k_tempx > k_default
            ki = k_default;
        end
    end
end

k = ki;
time_prec = time;
end

== matlab function dual_arm_1/Dual arm system/FRANKA_2/CORIOLIS ==
  data: q input; Fc output double; q_dot input
function Fc = fcn(q,q_dot)
coder.extrinsic('get_CoriolisMatrix');
C = zeros(7,7);
C = get_CoriolisMatrix(q,q_dot);

Fc = C*q_dot;

end

== matlab function dual_arm_1/Modulator2/k selection3 ==
  settings: updateMethod=DISCRETE
  data: time input; e_pos input; k output; F_ext input; F_max parameter; F_int_max parameter; k_default parameter; pos input; phase input; inc parameter; a0 parameter; berta parameter; csi parameter; mass parameter
function k = fcn(time,e_pos,F_ext,F_max, F_int_max,k_default,pos,phase,inc,a0, berta, csi,mass)

%% Description: Modulate stiffness and damping consequently of the admittance controller.
%%Inputs:     e_pos = position error 
%             F_ext = external force on EE
%             phase = flag acknowledging the current desired trajectory phase
%%Outputs:    k = value of stiffnes on single d.o.f
%%Parameters: F_max = treshold of disturbance
%             F_int_max = maximum interaction force
%             k_default = default value of stiffness
%             a0,berta,csi = parameters from stability conditions
%             mass = apparent mass

%% Initialization
persistent ki int time_prec

% persistent initialization
if isempty(ki)
    ki = k_default;
end

if isempty(int)
    int = 1000;
end

if isempty(time_prec)
    time_prec = 0;
end


%% Compute k
if phase == 0
    if abs(F_ext) > F_max %contact is detected
        ki = 0.995*ki; %arbitrarly decrease k 
        if int == 1000 %contact position not set yet
            int = pos;
        end
        % if interaction force is higher than threshold
        if ki*abs(e_pos) > F_int_max
            % set k
            ktemp_x = F_int_max/abs(e_pos);
            if ktemp_x < ki
                ki = ktemp_x;
            end
        end
    end
else
    if pos > int + 0.005 %safe to increase k
        k_dot = berta*(4*a0*sqrt(ki/mass)*(ki)^(3/2))/(sqrt(ki) + 2*a0*csi*sqrt(ki)); %maximum variation within stability conditions 
        k_tempx = ki + k_dot*(time -time_prec);
        %ki = inc*ki;
        ki = k_tempx;
        %if ki > k_default
        if k_tempx > k_default
            ki = k_default;
        end
    end
end

k = ki;
time_prec = time;
end

== matlab function dual_arm_1/Modulator2/retrieve error ==
  data: x input; e_pos output; x_des input
function e_pos = fcn(x,x_des)
%% trial: use error definition to change gains??
coder.extrinsic('DQ','D','ctranspose','translation','vec8','vec4','mtimes');

%% Initialize
xe = zeros(8,1);
e = zeros(4,1);
e_pos = zeros(3,1);

%% Compute position error
xe = vec8(DQ(x)'* DQ(x_des)); %pose displacement
%xe = re+0.5*eps*(pe*re)
%log(xe) = 0.5*phi*ne + 0.5*eps*pe
e = vec4(2*D(log(DQ(xe)))); %position error
e_pos = [e(2); e(3); e(4)];

end

== matlab function dual_arm_1/TRAJECTORY1_jerk2/2Dq ==
  data: xd input; x_des output; dxd input; ddxd input; r0 input; dx_des output; ddx_des output
function [x_des,dx_des,ddx_des] =  DQ(xd,dxd,ddxd,r0)
coder.extrinsic('DQ','vec8','vec6','vec4','P','D','translation','rotation_angle','rotation_axis','plus','minus','mtimes','log','exp');
%% Compute trajectory within dual quaternion domain
%initialization
x_des = zeros(8,1); 
dx_des = zeros(8,1); 
ddx_des = zeros(8,1); 
E = DQ([0,0,0,0,1,0,0,0]);
%dual quaternion trajectory
x_des = vec8(DQ(r0) + 0.5*E*(DQ(xd)*DQ(r0)));
dx_des =  vec8(0.5*E*(DQ(dxd)*DQ(r0)));
ddx_des = vec8(0.5*E*(DQ(ddxd)*DQ(r0)));
end

== matlab function dual_arm_1/TRAJECTORY1_jerk2/MATLAB Function1 ==
  data: t output; pos_i output; pos_f output; tf output; r0 output; x_in input; time input
function [t,pos_i,pos_f,tf,r0] = fcn(x_in,time)
coder.extrinsic('DQ','vec4','P','D','translation','rotation_angle','rotation_axis');
%initialization
pos_i = zeros(3,1);
pos_f = zeros(3,1);
tf = 0;
p0 = zeros(4,1);
r0 = zeros(4,1);
%retrieve intial EE pose
p0 = vec4(translation(DQ(x_in)));
pos_i = [p0(2);p0(3);p0(4)];
r0 = vec4(P(DQ(x_in)));

if (time>=0 && time<1) %go down
    pos_f = pos_i + [0;0;-0.2];
    tf = 1;
    t = time;
elseif (time>=1 && time<1.3) %pause
    pos_i = [p0(2);p0(3);p0(4)-0.2];
    pos_f = pos_i;
    tf = 0.3;
    t = time - 1;
elseif (time >= 1.3 && time < 2.3) %go up
    pos_i = [p0(2);p0(3);p0(4)-0.2];
    pos_f = pos_i + [0;0;0.2];
    tf = 1;
    t = time - 1.3;
else
    pos_i = [p0(2);p0(3);p0(4)];
    pos_f = pos_i;
    tf = 1000;
    t = time - 2.3;
end

== matlab function dual_arm_1/TRAJECTORY1_jerk2/compute desired trajectory ==
  data: t input; xd output; pos_i input; pos_f input; tf input; dxd output; ddxd output
function [xd,dxd,ddxd] = traj(t,pos_i,pos_f,tf)
%% description: compute minimum jerk trajectory
%inputs: t = time
%        pos_i = initial position
%        pos_f = final position
%        tf = desired time frame for trajectory
%outpus: xd,dxd,ddxd desired position,velocity and acceleration
xd = pos_i + (pos_i - pos_f)*(15*(t/tf)^4 - 6*(t/tf)^5 -10*(t/tf)^3);
dxd = (pos_i - pos_f)*(60*(t^3)/(tf^4) - 30*(t^4)/(tf^5) -30*(t^2)/(tf^3));
ddxd = (pos_i - pos_f)*(180*(t^2)/(tf^4) - 120*(t^3)/(tf^5) -60*(t)/(tf^3));

end

== matlab function dual_arm_1/Dual arm system/FRANKA_2/GRAVITY ==
  data: q input; G output double
function G = fcn(q)
coder.extrinsic('get_GravityVector');
G = zeros(7,1);
G = get_GravityVector(q);

end

== matlab function dual_arm_1/Dual arm system/FRANKA_2/Joint Friction ==
  data: q_dot input; tau_f output
function tau_f = fcn(q_dot)
coder.extrinsic('get_FrictionTorque');
tau_f = zeros(7,1);
tau_f = get_FrictionTorque(q_dot);

end

== matlab function dual_arm_1/Dual arm system/FRANKA_2/Joint Friction1 ==
  data: q_dot input; tau_f output
function tau_f = fcn(q_dot)
D=eye(7)*1;
tau_f = -D*q_dot;

end

== matlab function dual_arm_1/Dual arm system/FRANKA_2/MASS^-1 ==
  data: q input; ddq output; F_tot input double
function ddq = fcn(q,F_tot)
coder.extrinsic('get_MassMatrix');
B = zeros(7,7);
B = get_MassMatrix(q);
B(isnan(B)) = 0;

ddq = B\F_tot;                      % Ftot*M^-1

end

== matlab function dual_arm_1/Dual arm system/FRANKA_2/MATLAB Function ==
  data: F input; F_ext output double; q input
function F_ext  = fcn(F,q)
coder.extrinsic('loadrobot','geometricJacobian');
franka_cfr = loadrobot("frankaEmikaPanda", "DataFormat","row");
%init
F_ext = zeros(7,1);
Jg1 = zeros(6,9);
%get numeric geometric jacobian
Jg1 = geometricJacobian(franka_cfr,[q',0,0],'panda_link8');
Jg = Jg1(:,1:7);
Jg = [Jg(4:6,:);Jg(1:3,:)]; 
F_ext = (Jg')*F;

end

== matlab function dual_arm_1/Dual arm system/FRANKA_2/MATLAB Function3 ==
  data: psi_ext input; tau_ext output double; q input; franka_dh_matrix parameter
function tau_ext = fcn(psi_ext,q,franka_dh_matrix)
%% Description: maps external wrench into joint-space
coder.extrinsic('DQ','vec8'); 
coder.extrinsic('pose_jacobian','fkm','DQ_SerialManipulator');             
franka = DQ_SerialManipulator(franka_dh_matrix,'modified'); 
%% initialization
G = zeros(8,8);
J = zeros(8,8);
Jg = zeros(6,7); %geometric jacobian
x_pose = zeros(8,1);
tau_ext = zeros(7,1); 
%% fkm
x_pose = vec8(fkm(franka,[q;0]));
J = pose_jacobian(franka,[q;0]);
J1 = J(:,1:7); 
G = getG(x_pose); %generalized dual jacobian
Ibar = [zeros(3,1), eye(3), zeros(3,1), zeros(3,3);...
        zeros(3,1), zeros(3,3), zeros(3,1), eye(3)]; 
Jg = Ibar*G*J1;
tau_ext = (Jg)'* psi_ext;
end

== matlab function dual_arm_1/fkm2 ==
  data: q input; xr_in output; xa_in output; franka_dh_matrix parameter; b1 parameter; b2 parameter
function [xr_in,xa_in] = FKM(q,franka_dh_matrix,b1,b2)
%forward kinematic models franka arms
coder.extrinsic('DQ','DQ_SerialManipulator','set_reference_frame','vec8'); 
coder.extrinsic('DQ_CooperativeDualTaskSpace','relative_pose','absolute_pose');
franka1 = DQ_SerialManipulator(franka_dh_matrix,'standard'); 
franka2 = DQ_SerialManipulator(franka_dh_matrix,'standard');
% set base reference
set_reference_frame(franka1,DQ(b1));
set_reference_frame(franka2,DQ(b2));

%Initialization
xr_in = zeros(8,1);
xa_in = zeros(8,1); 

%retrieve initial conditions 
two_arms =  DQ_CooperativeDualTaskSpace(franka1, franka2);
xr_in = vec8(relative_pose(two_arms,q)); %relative pose
xa_in = vec8(absolute_pose(two_arms,q)); %absolute pose

end

== matlab function dual_arm_1/fkm1 ==
  data: q input; dq input; xr output; xa output; franka_dh_matrix parameter; b1 parameter; b2 parameter; dxr output; dxa output
function [xr,xa,dxr,dxa] = FKM(q,dq,franka_dh_matrix,b1,b2)

%% Forward kinematic models CDTS dual-arm
coder.extrinsic('DQ','DQ_SerialManipulator','set_reference_frame','vec8'); 
coder.extrinsic('DQ_CooperativeDualTaskSpace','relative_pose','absolute_pose');
coder.extrinsic('relative_pose_jacobian','absolute_pose_jacobian')

%load robots
franka1 = DQ_SerialManipulator(franka_dh_matrix,'standard'); 
franka2 = DQ_SerialManipulator(franka_dh_matrix,'standard');
% set base reference
set_reference_frame(franka1,DQ(b1));
set_reference_frame(franka2,DQ(b2));

%Initialization
xr = zeros(8,1);
xa = zeros(8,1); 
dxr = zeros(8,1);
dxa = zeros(8,1); 
Jr = zeros(8,14);
Ja = zeros(8,14); 

%retrieve current poses 
two_arms =  DQ_CooperativeDualTaskSpace(franka1, franka2);
xr = vec8(relative_pose(two_arms,q)); %relative pose
xa = vec8(absolute_pose(two_arms,q)); %absolute pose

%compute jacobians
Jr = relative_pose_jacobian(two_arms,q);
Ja = absolute_pose_jacobian(two_arms,q); 

dxr = Jr*dq;
dxa = Ja*dq; 

end
